simulink model "PsiCtr1"  (Simulink 7.9)
settings: Solver=ode45  StartTime=0.0  StopTime=10.0  RelTol=1e-3
undefined symbols (not defined in the file or in its folder): sigbuilder_block
settings Model: Creator=userk  LastModifiedBy=userk

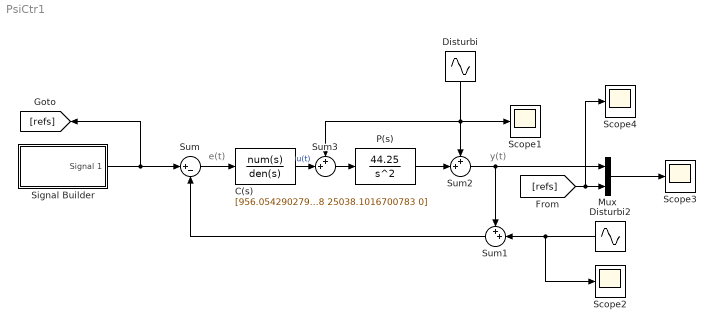
== system PsiCtr1 ==
  note: e(t)
  note: y(t)
  C(s) : TransferFcn  Numerator=[956.054290279666 33071.8047700315 165092.429920469 216024.761209075]  Denominator=[1 336.30408029458 25038.1016700783 0]
  Disturbi : Sin  Amplitude=0.003  Frequency=50  Phase=1  SampleTime=0
  Disturbi2 : Sin  Amplitude=0.003  Frequency=50  Phase=1  SampleTime=0
  Mux : Mux  Inputs=2
  P(s) : TransferFcn  Numerator=44.25  Denominator=[1 0 0]
  Scope{1..4} (4 alike) : Scope
      Scope2 settings: SaveName=ScopeData2
      Scope4 settings: SaveName=ScopeData3
  Signal Builder : Subsystem  Tag=STV Subsys  LoadFcn=sigbuilder_block('load');  StartFcn=sigbuilder_block('start');  StopFcn=sigbuilder_block('stop');  ClipboardFcn=sigbuilder_block('clipboard');  mask(Sigbuilder block){}
      mask help: Simulink:masks:SigbuilderBlock_MD
      mask init:
      | if ~strcmp(get_param(bdroot(gcbh),'SimulationStatus'),'stopped') tuvar = sigbuilder_block('maskInit'); end
      settings: CopyFcn=sigbuilder_block('copy');  DeleteFcn=sigbuilder_block('delete');  ModelCloseFcn=sigbuilder_block('modelClose');  PreSaveFcn=sigbuilder_block('preSave');  PauseFcn=sigbuilder_block('pause');  ContinueFcn=sigbuilder_block('continue');  NameChangeFcn=sigbuilder_block('namechange');  OpenFcn=sigbuilder_block('open',[397.6 120.8 550.4 400 ]);  CloseFcn=sigbuilder_block('close');
      mask Display: plot(0, 0, 100, 100,[2, 2, 32, 32, 2], [68, 8, 8, 68, 68],[32, 2], [38, 38], [32, 19, 2],[53, 60, 44], [32, 17, 17, 2],[16, 16, 31, 31]);txt = getActiveGroup(gcbh);text(2, 100, txt,'verticalAlignment', 'top');
  Sum : Sum  Inputs=|+-
  Sum1 : Sum  Inputs=++|
  Sum2 : Sum  Inputs=++|
  Sum3 : Sum  Inputs=++|
  wires:
  Sum/1 -> C(s)/1
  Disturbi/1 -> Sum2/1, Scope1/1, Sum3/1
  P(s)/1 -> Sum2/2
  Sum2/1 -> Sum1/1, Mux/1
  Sum1/1 -> Sum/2
  Signal Builder/1(Signal 1) -> Sum/1, [refs]
  [refs] -> Mux/2, Scope4/1
  Mux/1 -> Scope3/1
  Disturbi2/1 -> Sum1/2, Scope2/1
  Sum3/1 -> P(s)/1
  C(s)/1 -> Sum3/2  "u(t)"

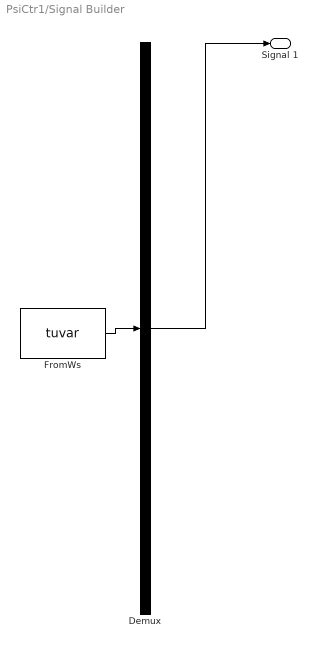
== system PsiCtr1/Signal Builder ==
  Demux : Demux  Tag=STV Demux  Outputs=1
  FromWs : FromWorkspace  Tag=STV FromWs  VariableName=tuvar  SampleTime=0  SigBuilderData=DataTag0  VnvData=DataTag1
      SigBuilderData=|
      | common.afterFinalStr = 'Extrapolate'
      | common.sampleTime = 0
      | dataSet.timeRange = [0 10]
      | dataSet.name = 'Group 1'
      | sbobj.Groups.Name = 'Group 1'
      | sbobj.Groups.Signals.Name = 'Signal 1'
      | sbobj.Groups.Signals.XData = [0 4.06 4.06 6 6 10]
      | sbobj.Groups.Signals.YData = [0 0.21 1 1 0.995 0.405]
  Signal 1 : Outport  Tag=STV Outport
  wires:
  Demux/1 -> Signal 1/1
  FromWs/1 -> Demux/1
